simulink library "Kl_SimuNIBoard"  (Simulink 7.8)
settings: Solver=ode5  SolverMode=SingleTasking  StartTime=0.0  StopTime=Inf  FixedStep=0.001  RelTol=1e-3
libraries: KL_SimuDI x1, KL_SimuDO x1, NI_Board_AI x1, NI_Board_AO x1, NiCiDuty x1
settings Model: Creator=Administrator  LastModifiedBy=Administrator

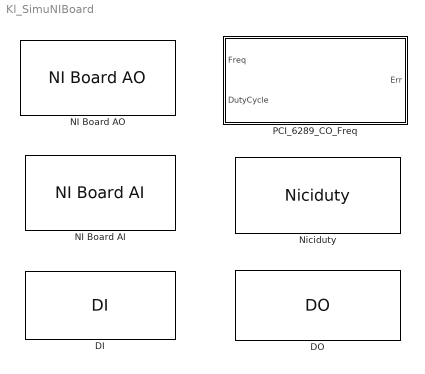
== system Kl_SimuNIBoard ==
  DI : KL_SimuDI/DI  nDev=1  nPort=1  nLine=0  nLineSelect=MultiLine  nStartLine=0  nEndLine=7
  DO : KL_SimuDO/DO  nDev=1  nPort=1  nLine=0  nLineSelect=MultiLine  nStartLine=0  nEndLine=7
  NI Board AI : NI_Board_AI/NI Board AI  nCon=0  nDev=0  nChan=0  nMode=DAQmx_Val_RSE  nMax=10  nMin=-10  nSamp=0  nReserve=0
  NI Board AO : NI_Board_AO/NI Board AO  nCon=0  nDev=1  nChan=0  nMax=10  nMin=-10  nSample=1  nReserve=0
  Niciduty : NiCiDuty/Niciduty  devid=0  chanid=0
  PCI_6289_CO_Freq : Subsystem  mask(NI_PCI_6289 For Counter Output){nDev=0, nChan=0, initialDelay=0}
      mask prompts: nDev "Dev ID:"; nChan "Chan ID:"; initialDelay "Delay Time:"
      mask help:
      | This block is used for CO.
      | You can specify the counter which you want to use.
      |
      | Block Parameters
      | Dev ID
      |     You can find the ID by nilsdev commond after you install DAQmx.
      | Chan ID
      |     Specify counter which you want to use.
      | Delay Time
      |     The amount of time in seconds to wait before generating the first pulse.
      | Err
      |     It will be -1 when a error occur.
      | DutyCycle
      |     The width of the pulse divided by the pulse period .
      | Freq
      |     The frequency at which to generate pulses .
      mask init:
      | displayblock=sprintf('\nPCI 6289 CO Frequency\nDev ID: %d Chan ID: %d\nDelay Time: %.2f\n', nDev, nChan,initialDelay);
      mask Help: You must Install The DAQmx of NI before you use it.You can find in Driver Dir.And there is a INSTALL file that will help you install it.
      mask Display: disp(displayblock);

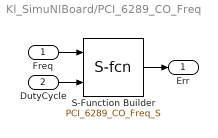
== system Kl_SimuNIBoard/PCI_6289_CO_Freq ==
  Freq : Inport
  DutyCycle : Inport  Port=2
  S-Function Builder : S-Function  InitFcn=try, set_param(gcb,'FunctionName','PCI_6289_CO_Freq_S'), end  FunctionName=PCI_6289_CO_Freq_S  Parameters=nDev,nChan,initialDelay  WizardData=DataTag0  EnableBusSupport=off  mask(S-Function Builder){}
      mask help: The S-Function Builder block creates a wrapper C-MEX S-function from your supplied C code with multiple input ports, output ports, and a variable number of scalar, vector, or matrix parameters. The input and output ports can propagate Simulink built-in data types, fixed-point datatypes, complex, frame, 1-D, and 2-D signals. This block also supports discrete and continuous states of type real. You can optionally have the block generate a TLC file to be used with Real-Time Workshop for code generation.
      mask init:
      | val = [[.9  0.75 0.75 1 1 .9 .9 1]',[1 1 0.75 0.75 .9 .9 1 .9]'];try , sys = get_param(gcb,'SfunBuilderFcnName');if isempty(sys), sys = get_param(gcb,'FunctionName'); end,catch, sys = get_param(gcb,'FunctionName'); end
      settings: CopyFcn=set_param(gcbh,'LinkStatus','none')  PreSaveFcn=try, set_param(gcb,'FunctionName','PCI_6289_CO_Freq_S'), end  OpenFcn=sfunctionwizard(gcbh)
      mask Display: plot(val(:,1),val(:,2)),disp(sys)port_label('input',1,'u0')port_label('input',2,'u1')port_label('output',1,'y0')
  Err : Outport
  wires:
  DutyCycle/1 -> S-Function Builder/2
  S-Function Builder/1 -> Err/1
  Freq/1 -> S-Function Builder/1
